simulink model "Simple_Quadcopter_Model_Sim_X_Yaw"  (R2017b)
settings: Solver=VariableStepAuto  StartTime=0.0  StopTime=TF  FixedStep=.001  RelTol=1e-3
values from neighbouring files (symbols this model uses):
  Ax = 0.0    (= 0)    [Simple_Quadcopter_model_Script_X_Yaw.m]
  Ay = 0.0    (= 0)    [Simple_Quadcopter_model_Script_X_Yaw.m]
  b = 1.144e-08    [Simple_Quadcopter_model_Script_X_Yaw.m]
  d = 9.94e-10    [Simple_Quadcopter_model_Script_X_Yaw.m]
  g = 9.81    [Simple_Quadcopter_model_Script_X_Yaw.m]
  Ixx = 7.5*10^(-3)    (= 0.0075)    [Simple_Quadcopter_model_Script_X_Yaw.m]
  Iyy = 7.5*10^(-3)    (= 0.0075)    [Simple_Quadcopter_model_Script_X_Yaw.m]
  Izz = 1.3*10^(-2)    (= 0.013)    [Simple_Quadcopter_model_Script_X_Yaw.m]
  Jr = 6.5*10^(-7)    (= 6.5e-07)    [Simple_Quadcopter_model_Script_X_Yaw.m]
  l = 0.1    [Simple_Quadcopter_model_Script_X_Yaw.m]
  m = weight/g    (= 0.0289500509684)    [Simple_Quadcopter_model_Script_X_Yaw.m]
settings Model: Creator=Nicky  LastModifiedBy=Nicky
settings CodeAppCC: StateflowObjectComments=on
settings SimscapeCC: SimscapeNormalizeSystem=off

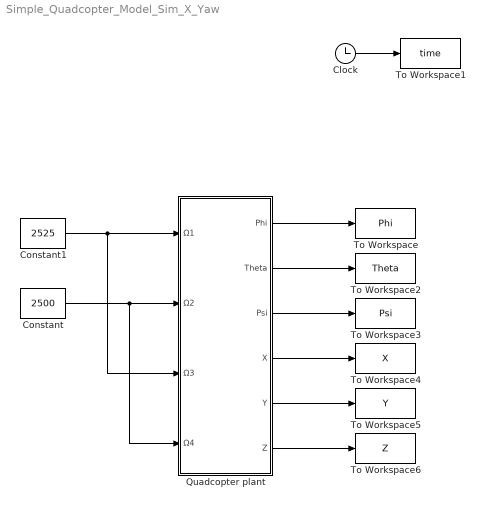
== system Simple_Quadcopter_Model_Sim_X_Yaw ==
  Clock : Clock
  Constant : Constant  Value=2500
  Constant1 : Constant  Value=2525
  Quadcopter plant : Subsystem
  To Workspace : ToWorkspace  VariableName=Phi  SampleTime=-1
      settings: Save2DSignal=2-D array (concatenate along first dimension)
  To Workspace1 : ToWorkspace  VariableName=time  SampleTime=-1
      settings: Save2DSignal=2-D array (concatenate along first dimension)
  To Workspace2 : ToWorkspace  VariableName=Theta  SampleTime=-1
      settings: Save2DSignal=2-D array (concatenate along first dimension)
  To Workspace3 : ToWorkspace  VariableName=Psi  SampleTime=-1
      settings: Save2DSignal=2-D array (concatenate along first dimension)
  To Workspace4 : ToWorkspace  VariableName=X  SampleTime=-1
      settings: Save2DSignal=2-D array (concatenate along first dimension)
  To Workspace5 : ToWorkspace  VariableName=Y  SampleTime=-1
      settings: Save2DSignal=2-D array (concatenate along first dimension)
  To Workspace6 : ToWorkspace  VariableName=Z  SampleTime=-1
      settings: Save2DSignal=2-D array (concatenate along first dimension)
  wires:
  Clock/1 -> To Workspace1/1
  Quadcopter plant/1(Phi) -> To Workspace/1
  Quadcopter plant/2(Theta) -> To Workspace2/1
  Quadcopter plant/3(Psi) -> To Workspace3/1
  Quadcopter plant/4(X) -> To Workspace4/1
  Quadcopter plant/5(Y) -> To Workspace5/1
  Quadcopter plant/6(Z) -> To Workspace6/1
  Constant1/1 -> Quadcopter plant/3(Ω3), Quadcopter plant/1(Ω1)
  Constant/1 -> Quadcopter plant/2(Ω2), Quadcopter plant/4(Ω4)

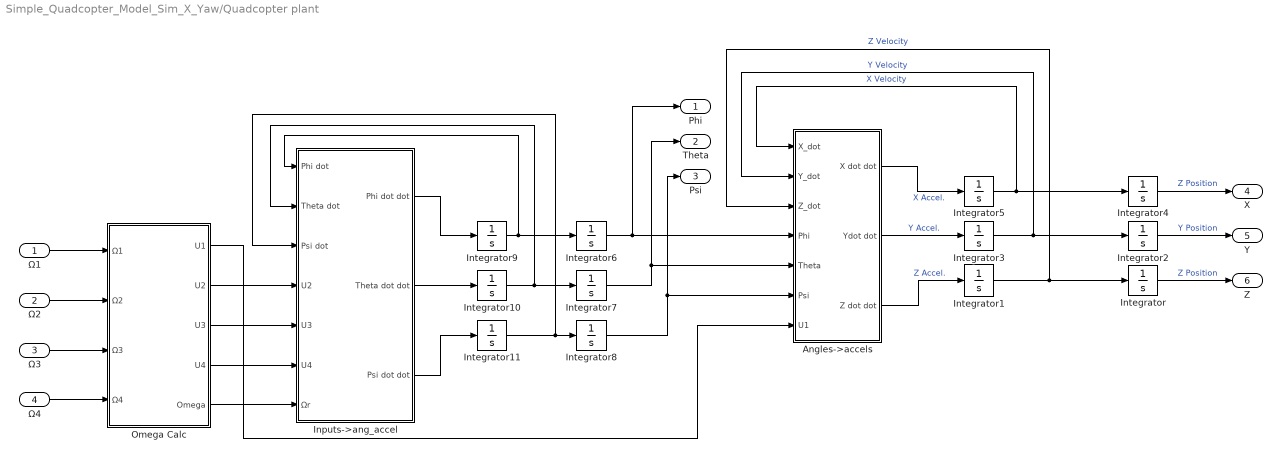
== system Simple_Quadcopter_Model_Sim_X_Yaw/Quadcopter plant ==
  Ω1 : Inport
  Ω2 : Inport  Port=2
  Ω3 : Inport  Port=3
  Ω4 : Inport  Port=4
  Angles->accels : Subsystem
  Inputs->ang_accel : Subsystem
  Integrator : Integrator  LimitOutput=on  UpperSaturationLimit=0
  Integrator{1..5,8..9} (7 alike) : Integrator
  Integrator10 : Integrator  UpperSaturationLimit=10000  LowerSaturationLimit=-10000
  Integrator11 : Integrator  UpperSaturationLimit=10000  LowerSaturationLimit=-10000
  Integrator6 : Integrator  WrapState=on
  Integrator7 : Integrator  WrapState=on
  Omega Calc : Subsystem
  Phi : Outport
  Theta : Outport  Port=2
  Psi : Outport  Port=3
  X : Outport  Port=4
  Y : Outport  Port=5
  Z : Outport  Port=6
  wires:
  Integrator1/1 -> Angles->accels/3(Z_dot), Integrator/1  "Z Velocity"
  Integrator2/1 -> Y/1  "Y Position"
  Integrator3/1 -> Angles->accels/2(Y_dot), Integrator2/1  "Y Velocity"
  Angles->accels/2(Ydot dot) -> Integrator3/1  "Y Accel."
  Angles->accels/3(Z dot dot) -> Integrator1/1  "Z Accel."
  Integrator8/1 -> Angles->accels/6(Psi), Psi/1
  Integrator7/1 -> Angles->accels/5(Theta), Theta/1
  Integrator6/1 -> Angles->accels/4(Phi), Phi/1
  Integrator11/1 -> Inputs->ang_accel/3(Psi dot), Integrator8/1
  Integrator10/1 -> Inputs->ang_accel/2(Theta dot), Integrator7/1
  Integrator9/1 -> Inputs->ang_accel/1(Phi dot), Integrator6/1
  Inputs->ang_accel/2(Theta dot dot) -> Integrator10/1
  Inputs->ang_accel/1(Phi dot dot) -> Integrator9/1
  Inputs->ang_accel/3(Psi dot dot) -> Integrator11/1
  Omega Calc/5(Omega) -> Inputs->ang_accel/7(Ωr)
  Omega Calc/4(U4) -> Inputs->ang_accel/6(U4)
  Omega Calc/3(U3) -> Inputs->ang_accel/5(U3)
  Omega Calc/2(U2) -> Inputs->ang_accel/4(U2)
  Omega Calc/1(U1) -> Angles->accels/7(U1)
  Ω2/1 -> Omega Calc/2(Ω2)
  Ω3/1 -> Omega Calc/3(Ω3)
  Ω4/1 -> Omega Calc/4(Ω4)
  Integrator/1 -> Z/1  "Z Position"
  Integrator5/1 -> Angles->accels/1(X_dot), Integrator4/1  "X Velocity"
  Angles->accels/1(X dot dot) -> Integrator5/1  "X Accel."
  Integrator4/1 -> X/1  "Z Position"
  Ω1/1 -> Omega Calc/1(Ω1)

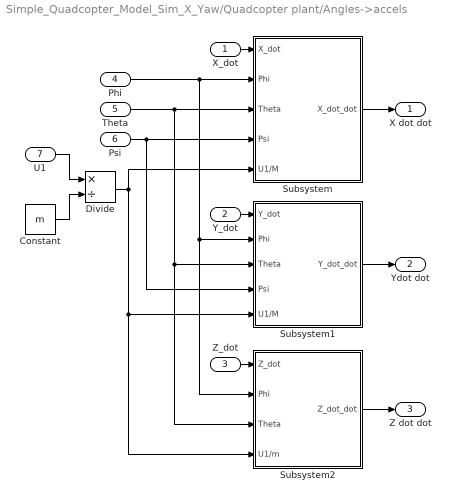
== system Simple_Quadcopter_Model_Sim_X_Yaw/Quadcopter plant/Angles->accels ==
  X_dot : Inport
  Y_dot : Inport  Port=2
  Z_dot : Inport  Port=3
  Phi : Inport  Port=4
  Theta : Inport  Port=5
  Psi : Inport  Port=6
  U1 : Inport  Port=7
  Constant : Constant  Value=m
  Divide : Product  Inputs=*/
  Subsystem : Subsystem
  Subsystem1 : Subsystem
  Subsystem2 : Subsystem
  X dot dot : Outport
  Ydot dot : Outport  Port=2
  Z dot dot : Outport  Port=3
  wires:
  Phi/1 -> Subsystem2/2(Phi), Subsystem1/2(Phi), Subsystem/2(Phi)
  U1/1 -> Divide/1
  Constant/1 -> Divide/2
  Divide/1 -> Subsystem/5(U1/M), Subsystem2/4(U1/m), Subsystem1/5(U1/M)
  Subsystem/1(X_dot_dot) -> X dot dot/1
  Subsystem1/1(Y_dot_dot) -> Ydot dot/1
  Subsystem2/1(Z_dot_dot) -> Z dot dot/1
  Theta/1 -> Subsystem2/3(Theta), Subsystem1/3(Theta), Subsystem/3(Theta)
  Psi/1 -> Subsystem1/4(Psi), Subsystem/4(Psi)
  X_dot/1 -> Subsystem/1(X_dot)
  Y_dot/1 -> Subsystem1/1(Y_dot)
  Z_dot/1 -> Subsystem2/1(Z_dot)

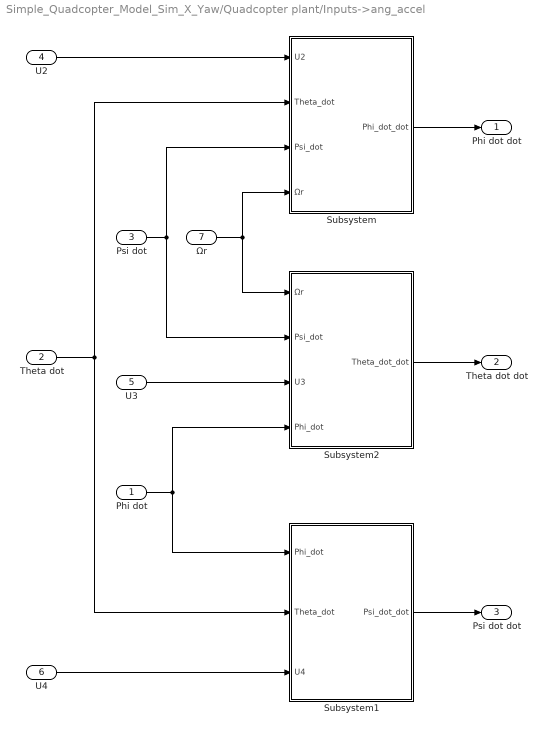
== system Simple_Quadcopter_Model_Sim_X_Yaw/Quadcopter plant/Inputs->ang_accel ==
  Phi dot : Inport
  Theta dot : Inport  Port=2
  Psi dot : Inport  Port=3
  U2 : Inport  Port=4
  U3 : Inport  Port=5
  U4 : Inport  Port=6
  Ωr : Inport  Port=7
  Subsystem : Subsystem
  Subsystem1 : Subsystem
  Subsystem2 : Subsystem
  Phi dot dot : Outport
  Theta dot dot : Outport  Port=2
  Psi dot dot : Outport  Port=3
  wires:
  U3/1 -> Subsystem2/3(U3)
  U4/1 -> Subsystem1/3(U4)
  Subsystem/1(Phi_dot_dot) -> Phi dot dot/1
  U2/1 -> Subsystem/1(U2)
  Ωr/1 -> Subsystem/4(Ωr), Subsystem2/1(Ωr)
  Psi dot/1 -> Subsystem2/2(Psi_dot), Subsystem/3(Psi_dot)
  Subsystem2/1(Theta_dot_dot) -> Theta dot dot/1
  Subsystem1/1(Psi_dot_dot) -> Psi dot dot/1
  Theta dot/1 -> Subsystem/2(Theta_dot), Subsystem1/2(Theta_dot)
  Phi dot/1 -> Subsystem2/4(Phi_dot), Subsystem1/1(Phi_dot)

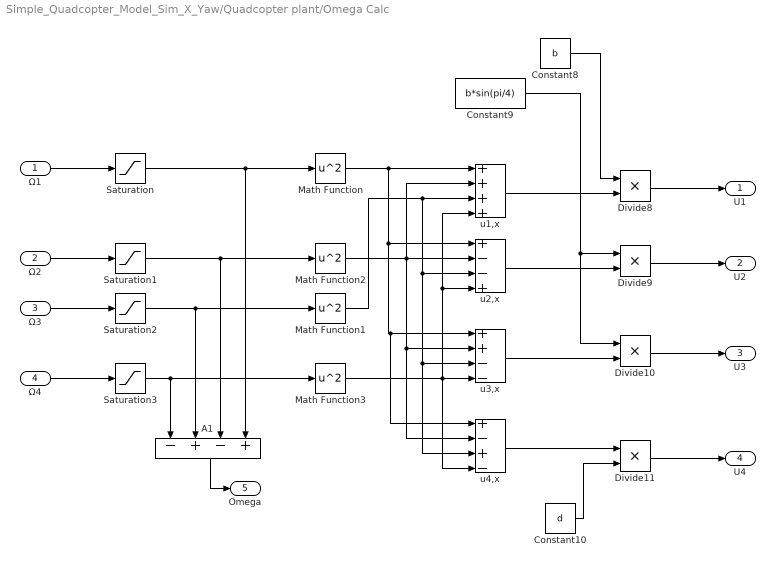
== system Simple_Quadcopter_Model_Sim_X_Yaw/Quadcopter plant/Omega Calc ==
  Ω1 : Inport
  Ω2 : Inport  Port=2
  Ω3 : Inport  Port=3
  Ω4 : Inport  Port=4
  A1 : Sum  Inputs=-+-+
  Constant10 : Constant  Value=d
  Constant8 : Constant  Value=b
  Constant9 : Constant  Value=b*sin(pi/4)
  Divide{8..11} (4 alike) : Product  Inputs=**
  Math Function{,1..3} (4 alike) : Math  Operator=square  SaturateOnIntegerOverflow=on
  Saturation{,1..3} (4 alike) : Saturate  UpperLimit=inf  LowerLimit=0
  u1,x : Sum  Inputs=++++
  u2,x : Sum  Inputs=+--+
  u3,x : Sum  Inputs=++--
  u4,x : Sum  Inputs=+-+-
  U1 : Outport
  U2 : Outport  Port=2
  U3 : Outport  Port=3
  U4 : Outport  Port=4
  Omega : Outport  Port=5
  wires:
  Constant10/1 -> Divide11/2
  u4,x/1 -> Divide11/1
  u3,x/1 -> Divide10/2
  u2,x/1 -> Divide9/2
  Constant9/1 -> Divide10/1, Divide9/1
  u1,x/1 -> Divide8/2
  Constant8/1 -> Divide8/1
  A1/1 -> Omega/1
  Divide8/1 -> U1/1
  Divide9/1 -> U2/1
  Divide10/1 -> U3/1
  Divide11/1 -> U4/1
  Math Function/1 -> u4,x/1, u3,x/1, u2,x/1, u1,x/1
  Math Function1/1 -> u4,x/3, u3,x/3, u2,x/3, u1,x/3
  Math Function2/1 -> u1,x/2, u4,x/2, u3,x/2, u2,x/2
  Math Function3/1 -> u1,x/4, u2,x/4, u4,x/4, u3,x/4
  Ω1/1 -> Saturation/1
  Ω2/1 -> Saturation1/1
  Ω3/1 -> Saturation2/1
  Ω4/1 -> Saturation3/1
  Saturation2/1 -> A1/2, Math Function1/1
  Saturation1/1 -> Math Function2/1, A1/3
  Saturation/1 -> Math Function/1, A1/4
  Saturation3/1 -> A1/1, Math Function3/1

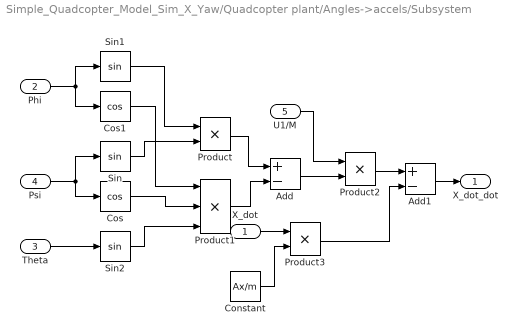
== system Simple_Quadcopter_Model_Sim_X_Yaw/Quadcopter plant/Angles->accels/Subsystem ==
  X_dot : Inport
  Phi : Inport  Port=2
  Theta : Inport  Port=3
  Psi : Inport  Port=4
  U1/M : Inport  Port=5
  Add : Sum  Inputs=+-
  Add1 : Sum  Inputs=+-
  Constant : Constant  Value=Ax/m
  Cos : Trigonometry  Operator=cos
  Cos1 : Trigonometry  Operator=cos
  Product : Product
  Product1 : Product  Inputs=3
  Product2 : Product
  Product3 : Product
  Sin : Trigonometry
  Sin1 : Trigonometry
  Sin2 : Trigonometry
  X_dot_dot : Outport
  wires:
  Product1/1 -> Add/2
  Product/1 -> Add/1
  U1/M/1 -> Product2/1
  Add/1 -> Product2/2
  Psi/1 -> Cos/1, Sin/1
  Phi/1 -> Cos1/1, Sin1/1
  Theta/1 -> Sin2/1
  Cos1/1 -> Product1/1
  Cos/1 -> Product1/2
  Sin2/1 -> Product1/3
  Sin1/1 -> Product/1
  Sin/1 -> Product/2
  Product2/1 -> Add1/1
  Add1/1 -> X_dot_dot/1
  X_dot/1 -> Product3/1
  Constant/1 -> Product3/2
  Product3/1 -> Add1/2

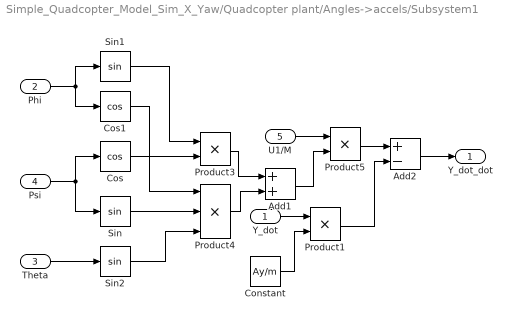
== system Simple_Quadcopter_Model_Sim_X_Yaw/Quadcopter plant/Angles->accels/Subsystem1 ==
  Y_dot : Inport
  Phi : Inport  Port=2
  Theta : Inport  Port=3
  Psi : Inport  Port=4
  U1/M : Inport  Port=5
  Add1 : Sum
  Add2 : Sum  Inputs=+-
  Constant : Constant  Value=Ay/m
  Cos : Trigonometry  Operator=cos
  Cos1 : Trigonometry  Operator=cos
  Product1 : Product
  Product3 : Product
  Product4 : Product  Inputs=3
  Product5 : Product
  Sin : Trigonometry
  Sin1 : Trigonometry
  Sin2 : Trigonometry
  Y_dot_dot : Outport
  wires:
  Psi/1 -> Sin/1, Cos/1
  Phi/1 -> Cos1/1, Sin1/1
  Theta/1 -> Sin2/1
  Add1/1 -> Product5/2
  Product4/1 -> Add1/2
  U1/M/1 -> Product5/1
  Product3/1 -> Add1/1
  Cos1/1 -> Product4/1
  Sin/1 -> Product4/2
  Sin2/1 -> Product4/3
  Sin1/1 -> Product3/1
  Cos/1 -> Product3/2
  Y_dot/1 -> Product1/1
  Constant/1 -> Product1/2
  Product1/1 -> Add2/2
  Product5/1 -> Add2/1
  Add2/1 -> Y_dot_dot/1

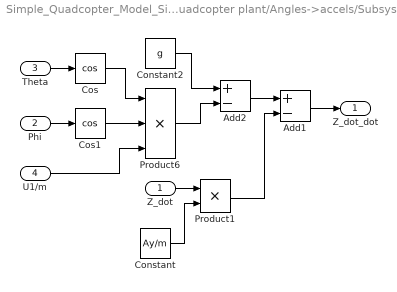
== system Simple_Quadcopter_Model_Sim_X_Yaw/Quadcopter plant/Angles->accels/Subsystem2 ==
  Z_dot : Inport
  Phi : Inport  Port=2
  Theta : Inport  Port=3
  U1/m : Inport  Port=4
  Add1 : Sum  Inputs=+-
  Add2 : Sum  Inputs=+-
  Constant : Constant  Value=Ay/m
  Constant2 : Constant  Value=g
  Cos : Trigonometry  Operator=cos
  Cos1 : Trigonometry  Operator=cos
  Product1 : Product
  Product6 : Product  Inputs=3
  Z_dot_dot : Outport
  wires:
  Phi/1 -> Cos1/1
  Theta/1 -> Cos/1
  U1/m/1 -> Product6/3
  Constant2/1 -> Add2/1
  Cos/1 -> Product6/1
  Product6/1 -> Add2/2
  Cos1/1 -> Product6/2
  Product1/1 -> Add1/2
  Z_dot/1 -> Product1/1
  Constant/1 -> Product1/2
  Add2/1 -> Add1/1
  Add1/1 -> Z_dot_dot/1

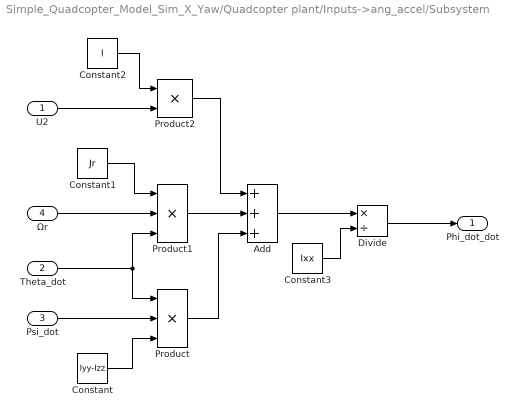
== system Simple_Quadcopter_Model_Sim_X_Yaw/Quadcopter plant/Inputs->ang_accel/Subsystem ==
  U2 : Inport
  Theta_dot : Inport  Port=2
  Psi_dot : Inport  Port=3
  Ωr : Inport  Port=4
  Add : Sum  Inputs=+++
  Constant : Constant  Value=Iyy-Izz
  Constant1 : Constant  Value=Jr
  Constant2 : Constant  Value=l
  Constant3 : Constant  Value=Ixx
  Divide : Product  Inputs=*/
  Product : Product  Inputs=3
  Product1 : Product  Inputs=3
  Product2 : Product
  Phi_dot_dot : Outport
  wires:
  Psi_dot/1 -> Product/2
  Theta_dot/1 -> Product/1, Product1/3
  Constant/1 -> Product/3
  Ωr/1 -> Product1/2
  Constant1/1 -> Product1/1
  U2/1 -> Product2/2
  Constant2/1 -> Product2/1
  Product1/1 -> Add/2
  Product2/1 -> Add/1
  Product/1 -> Add/3
  Add/1 -> Divide/1
  Constant3/1 -> Divide/2
  Divide/1 -> Phi_dot_dot/1

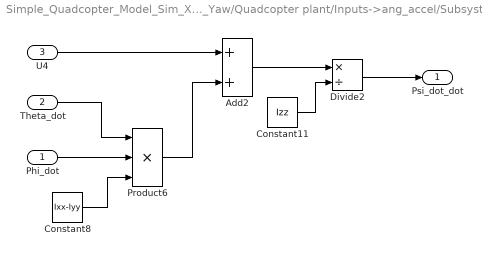
== system Simple_Quadcopter_Model_Sim_X_Yaw/Quadcopter plant/Inputs->ang_accel/Subsystem1 ==
  Phi_dot : Inport
  Theta_dot : Inport  Port=2
  U4 : Inport  Port=3
  Add2 : Sum
  Constant11 : Constant  Value=Izz
  Constant8 : Constant  Value=Ixx-Iyy
  Divide2 : Product  Inputs=*/
  Product6 : Product  Inputs=3
  Psi_dot_dot : Outport
  wires:
  Theta_dot/1 -> Product6/1
  Phi_dot/1 -> Product6/2
  Constant8/1 -> Product6/3
  Add2/1 -> Divide2/1
  Constant11/1 -> Divide2/2
  Divide2/1 -> Psi_dot_dot/1
  Product6/1 -> Add2/2
  U4/1 -> Add2/1

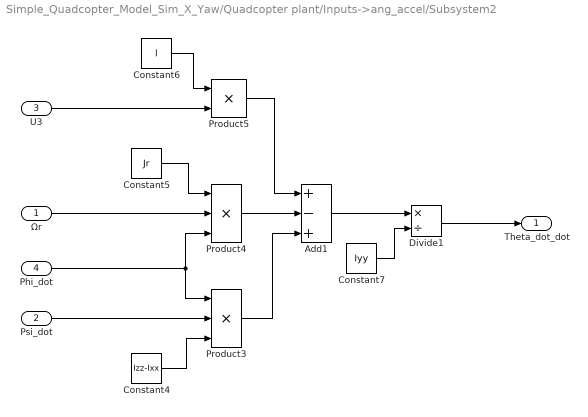
== system Simple_Quadcopter_Model_Sim_X_Yaw/Quadcopter plant/Inputs->ang_accel/Subsystem2 ==
  Ωr : Inport
  Psi_dot : Inport  Port=2
  U3 : Inport  Port=3
  Phi_dot : Inport  Port=4
  Add1 : Sum  Inputs=+-+
  Constant4 : Constant  Value=Izz-Ixx
  Constant5 : Constant  Value=Jr
  Constant6 : Constant  Value=l
  Constant7 : Constant  Value=Iyy
  Divide1 : Product  Inputs=*/
  Product3 : Product  Inputs=3
  Product4 : Product  Inputs=3
  Product5 : Product
  Theta_dot_dot : Outport
  wires:
  Psi_dot/1 -> Product3/2
  Phi_dot/1 -> Product3/1, Product4/3
  Ωr/1 -> Product4/2
  Constant4/1 -> Product3/3
  Constant5/1 -> Product4/1
  U3/1 -> Product5/2
  Constant6/1 -> Product5/1
  Product4/1 -> Add1/2
  Product5/1 -> Add1/1
  Product3/1 -> Add1/3
  Add1/1 -> Divide1/1
  Constant7/1 -> Divide1/2
  Divide1/1 -> Theta_dot_dot/1
